simulink library "DRC_SimulinkLibrary"  (R2024a)
settings: Solver=VariableStepAuto  StartTime=0.0  StopTime=10.0  RelTol=1e-3
values from neighbouring files (symbols this model uses):
  T = 0.5*rho*A*R*V^2*Cp/TSR    [aerodynamictorque.m]
undefined symbols (not defined in the file or in its folder): DiscIntNeverNeededParam, freq, maxSatValue, OmegaVector, Ts, Wr0, WSE
libraries: $bdroot x16, spsEdgeDetectorLib x1
settings Model: Creator=Sebastiaan  LastModifiedBy=glazzerini
settings DebuggingCC: UnconnectedInputMsg=warning  UnconnectedOutputMsg=warning  UnconnectedLineMsg=warning
settings ModelReferenceCC: EnableRefExpFcnMdlSchedulingChecks=on
settings RTWCC: GPUComputeCapability=3.5  DLArmComputeVersion=19.05

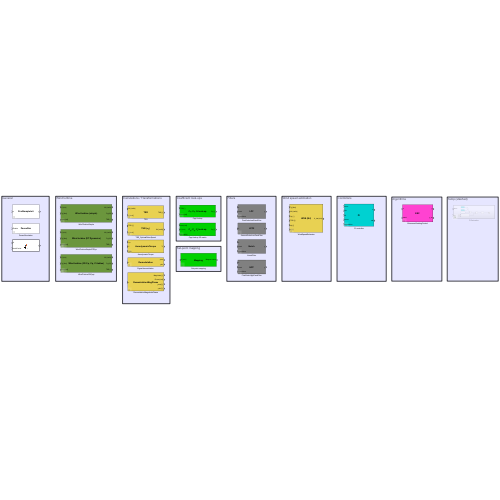
[thumbnail: Simulink's stored preview of the top-level diagram]
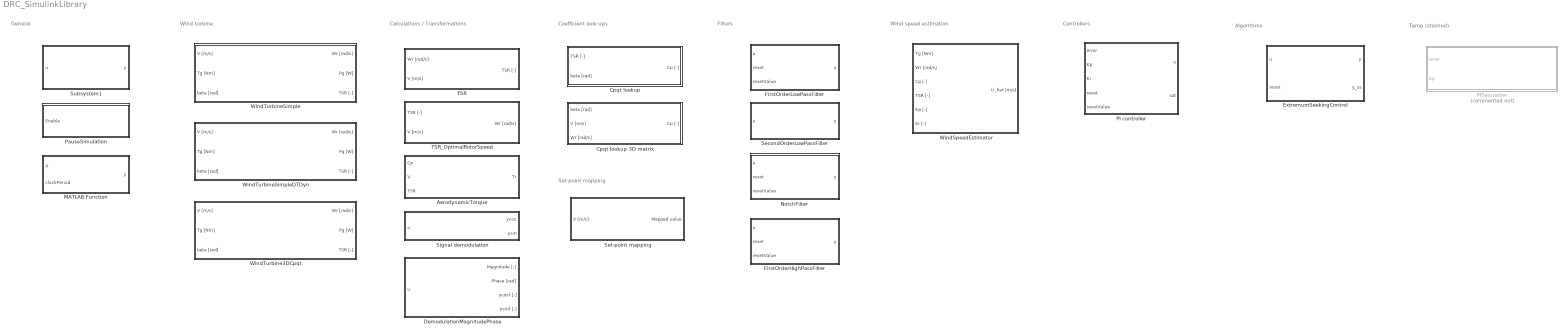
== system DRC_SimulinkLibrary ==
  note: Filters
  note: Coefficient look-ups
  note: General
  note: Algorithms
  note: Wind speed estimation
  note: Controllers
  note: Calculations / Transformations
  note: Temp (stashed)
  note: Wind turbine
  note: Set-point mapping
  AerodynamicTorque : Subsystem  mask(Aerodynamic rotor torque){R=10, rho=1.225, TrMax=inf}
      mask prompts: R "Rotor radius [m]"; rho "Air density [kg/m^3]"; TrMax "Maximum aerodynamic torque [Nm]"
      mask help: Calculates aerodynamic rotor torque based on the rotor radius, air density, power coefficient, wind speed and tip-speed ratio.
      mask Display: disp('{\bf\fontsize{12}AerodynamicTorque}', 'texmode', 'on');
  Cpqt lookup : Subsystem  mask(Coefficient look-up){CpqtGrid=[], TSRVector=[], PitchVector=[]}
      mask prompts: CpqtGrid "Cp/Cq/Ct grid [-]"; TSRVector "TSR vector [-]"; PitchVector "Pitch vector [rad]"
      mask help: Coefficient look-up table for power coefficient (Cp), torque coefficient (Cq), and thrust coefficient (Ct). The TSR and Pitch data should be a 1-dimensional vector of sizes p and q, respectively. The provided coefficient matrix should be of size p x q.
      mask Display: disp('{\bf\fontsize{12}C_p, C_q, C_t look-up}', 'texmode', 'on');
  Cpqt lookup 3D matrix : Subsystem  mask(Coefficient look-up){CpqtGrid=[], PitchVector=[], WindSpeedVector=[], OmegaVector=[]}
      mask prompts: CpqtGrid "Cp/Cq/Ct grid [-]"; PitchVector "Pitch vector [rad]"; WindSpeedVector "Wind Speed vector [m/s]"; OmegaVector "Omega vector [rad/s]"
      mask help: Coefficient look-up matrices for power coefficient (Cp), torque coefficient (Cq), and thrust coefficient (Ct). The Pitch, Wind-speed and Omega data should be 1-dimensional vectors of sizes p, q and r respectively. The provided coefficient matrix should be of size p x q x r.
      mask Display: disp('{\bf\fontsize{12}C_p, C_q, C_t look-up}', 'texmode', 'on');
  DemodulationMagnitudePhase : Subsystem  mask(Signal demodulation (mag/phase){freq=-1, phase_offset=0, Ts=-1, betaNum=0.1, betaDen=10}
      mask prompts: freq "Frequency [rad/s]"; phase_offset "Phase offset [rad]"; Ts "Sampling time [s]"; betaNum "Damping numerator"; betaDen "Damping denominator"
      mask help: This block demodulates a specific frequency in the input signal and returns its magnitude and phase. The input signal should have a zero-mean, which can for example be accomplished by high-pass or band-pass filtering.
      mask DialogControl Container3 Prompt: Notch parameters
      mask Display: disp('{\bf\fontsize{12}DemodulationMagPhase}', 'texmode', 'on');
  ExtremumSeekingControl : Subsystem  mask(Extremum Seeking Control (ESC)){D_A=3e5, D_w=0.09, M_phi=-30/180*pi, Ki=1000, LPF_wc=0.1, HPF_wc=0.02, Ts=Ts}
      mask prompts: D_A "Dither amplitude"; D_w "Dither frequency [rad/s]"; M_phi "Demodulation phase offset [rad]"; Ki "Integrator gain"; LPF_wc "LPF cut-off frequency [rad/s]"; HPF_wc "HPF cut-in frequency [rad/s]"; Ts "Sampling time [s]"
      mask help: Extremum Seeking Control (ESC) is a filter-based algorithm that excites a system with a periodic signal to attain a local maximum as a function of the input signal. By periodic excitation, demodulation and filtering actions the output gradient is retrieved, and subject to time integration until the steady-state signal that maximizes (or minimizes) the system output is attained.
      mask Display: disp('{\bf\fontsize{12}ESC}', 'texmode', 'on');
  FirstOrderHighPassFilter : Subsystem  mask(First order high-pass filter){wc=-1, Ts=-1}
      mask prompts: wc "Cut-off frequency [rad/s]"; Ts "Sampling time [s]"
      mask help:
      | Discrete time notch filter (IIR), given in continuous time by:
      | G =  s / (s + wc)
      | with wc the cut-off frequency, and s the Laplace operator.
      |
      | Discretized using the bilinear transform (Tustin's method). The sampling time should be explicitly specified.
      mask Display: disp('{\bf\fontsize{12}HPF}', 'texmode', 'on');
  FirstOrderLowPassFilter : Subsystem  mask(First order low-pass filter){wc=-1, Ts=-1}
      mask prompts: wc "Cut-in frequency [rad/s]"; Ts "Sampling time [s]"
      mask help:
      | Discrete time first order low-pass filter (IIR), given in continuous time by:
      | G = wc / ( s + wc)
      | with wc the cut-off frequency, and s the Laplace operator.
      |
      | Discretized using the bilinear transform (Tustin's method). The sampling time should be explicitly specified.
      mask Display: disp('{\bf\fontsize{12}LPF}', 'texmode', 'on');
  MATLAB Function : MATLAB Function  TreatAsAtomicUnit=on
  NotchFilter : Subsystem  mask{wn=-1, betaNum=-1, betaDen=-1, Ts=-1}
      mask prompts: wn "Target frequency [rad/s]"; betaNum "Beta numerator [-]"; betaDen "Beta denominator [-]"; Ts "Sampling time [s]"
      mask help:
      | Discrete time notch filter (IIR), given in continuous time by:
      | G =  ( s^2 + 2*wc*betaNum*s + wc^2 ) / ( s^2 + 2*wc*betaDen*s + wc^2 )
      | with wc the cut-off frequency, betaNum and betaDen being the damping coefficients, and s the Laplace operator. The ratio and magnitude of the ratio determines the width and depth of the notch.
      |
      | Discretized using the bilinear transform (Tustin's method). The sampling time should be explicitly specified.
      mask Display: disp('{\bf\fontsize{12}Notch}', 'texmode', 'on');
  PI controller : Subsystem  mask(PI controller){minSatValue=0, maxSatValue=inf, Ts=Ts}
      mask prompts: minSatValue "Minimum saturation"; maxSatValue "Maximum saturation"; Ts "Sampling time [s]"
      mask help:
      | Proportional-Integral (PI) controller with saturation limits. The error port is the input to the controller, Kp and Ki are the proportional and integral gains amplifying the error signal. When reset is true, the integral state is reset to resetValue.
      |
      | The sat output port indicates whether the controller is saturated or if the reset port is true.
      mask Display: disp('{\bf\fontsize{12}PI}', 'texmode', 'on');
  PISaturation : Subsystem  Commented=on
  PauseSimulation : Subsystem  mask(Pause simulation){PauseEach=0.5, Ts=Ts}
      mask prompts: PauseEach "Pause each [s]"; Ts "Sampling time [s]"
      mask help: Pause simulation after integer multiples of the specified value.
      mask Display: disp('{\bf\fontsize{12}PauseSim}', 'texmode', 'on');
  SecondOrderLowPassFilter : Subsystem  mask(Second order low-pass filter){wn=-1, damp=-1, Ts=-1}
      mask prompts: wn "Cut-off frequency [rad/s]"; damp "Damping coefficient [-]"; Ts "Sampling time [s]"
      mask help:
      | Discrete time second order low-pass filter (IIR), given in continuous time by:
      | G = wc^2 / ( s^2 + 2*wc*zeta*s + wc^2)
      | with wc the cut-off frequency, zeta the damping coefficient, and s the Laplace operator.
      |
      | Discretized using the bilinear transform (Tustin's method). The sampling time should be explicitly specified.
      mask Display: disp('{\bf\fontsize{12}LPF2}', 'texmode', 'on');
  Set-point mapping : Subsystem  mask(Mapping look-up){MappingVector=[], WindSpeedVector=[]}
      mask help: Mapping look-up for rotational speed or collective pitch angle vs windspeed. The input data should be a 1-dimensional value. The provided value will represent the mapping.
      mask Display: disp('{\bf\fontsize{12}Mapping}', 'texmode', 'on');
  "Signal demodulation " : Subsystem  mask(Signal demodulation){freq=freq, phase_offset=0, Ts=Ts}
      mask prompts: freq "Frequency [rad/s]"; phase_offset "Phase offset [rad]"; Ts "Sampling time [s]"
      mask help: This block demodulates a specific frequency in the input signal and returns the sine and cosine projections as output. The input signal should have a zero-mean, which can for example be accomplished by high-pass or band-pass filtering.
      mask Display: disp('{\bf\fontsize{12}Demodulation}', 'texmode', 'on');
  Subsystem1 : Subsystem  mask(First sample initialization){u_init=0}
      mask prompts: u_init "First sample"
      mask help: Returns the value specified by First sample in the very first time step. In subsequent time steps: y=u.
      mask Display: disp('{\bf\fontsize{12}FirstSampleInit}', 'texmode', 'on');
  TSR : Subsystem  mask(Tip-speed ratio){RotorRadius=10}
      mask prompts: RotorRadius "Rotor radius [m]"
      mask help: Calculates the tip-speed ratio based on rotor speed [rad/s] and wind speed [m/s] signals.
      mask Display: disp('{\bf\fontsize{12}TSR}', 'texmode', 'on');
  TSR_OptimalRotorSpeed : Subsystem  mask(Tip-speed ratio (rotor speed)){RotorRadius=10}
      mask prompts: RotorRadius "Rotor radius [m]"
      mask help: Calculates the corresponding rotor speed [rad/s] based on tip-speed ratio [-] and wind speed [m/s] signals.
      mask Display: disp('{\bf\fontsize{12}TSR (\omega_r)}', 'texmode', 'on');
  WindSpeedEstimator : Subsystem  mask(Wind speed estimator (I&I)){R=T.R, TrMax=T.Tgen_max*T.G, G=T.G, JLss=T.Jlss, rho=T.rho, omega_r_0=WSE.omega_r_0, V0=0, Ts=Ts}
      mask prompts: R "Rotor radius [m]"; TrMax "Max. exp. rotor torque [Nm]"; G "Gearbox ratio"; JLss "Drivetrain inertia (LSS)"; rho "Air density [kg/m^3]"; omega_r_0 "Rotor speed initial condition"; V0 "Wind speed initial condition"; Ts "Sampling time [s]"
      mask help: Immersion and Invariance (I&I) wind speed estimator. Uses prior power coefficient information of the turbine to obtain an estimate of the aerodynamic rotor torque. Together with the measured generator torque and rotor speed, an estimate of the wind speed is computed.
      mask Display: disp('{\bf\fontsize{12}WSE (I&I)}', 'texmode', 'on');
  WindTurbine3DCpqt : Subsystem  AncestorBlock=DRC_SimulinkLibrary/WindTurbineSimple  mask{R=T.R, rho=T.rho, TMax=inf, JWr=T.Jlss, G=T.G, Wr0=Wr0, CpArray=T.Cp, betaVec=T.CPitch, wsVec=T.CWindSpeed, omegaVec=T.COmega}
      mask prompts: R "Rotor radius [m]"; rho "Air density [kg/m^3]"; TMax "Maximum aerodynamic torque [Nm]"; JWr "Inertia low-speed shaft [kg m^2]"; G "Gearbox ratio [-]"; Wr0 "Rotor speed initial condition [rad/s]"; CpArray "Cp matrix"; betaVec "Pitch vector [rad]"; wsVec "Wind speed vector [m/s]"; omegaVec "Omega vector [rad/s]"
      mask DialogControl CpGroupVar Prompt: Power coefficient (Cp)
      mask Display: disp('{\bf\fontsize{12}Wind turbine (3D Cp, Cq, Ct tables)}', 'texmode', 'on');
  WindTurbineSimple : Subsystem  mask{R=T.R, rho=T.rho, TMax=inf, JWr=T.Jlss, G=T.G, Wr0=Wr0, CpArray=T.Cp, TSRVec=T.CTSR, betaVec=T.CPitch}
      mask prompts: R "Rotor radius [m]"; rho "Air density [kg/m^3]"; TMax "Maximum aerodynamic torque [Nm]"; JWr "Inertia low-speed shaft [kg m^2]"; G "Gearbox ratio [-]"; Wr0 "Rotor speed initial condition [rad/s]"; CpArray "Cp matrix"; TSRVec "Tip-speed ratio vector"; betaVec "Pitch vector [rad]"
      mask DialogControl CpGroupVar Prompt: Power coefficient (Cp)
      mask Display: disp('{\bf\fontsize{12}Wind turbine (simple)}', 'texmode', 'on');
  WindTurbineSimpleDTDyn : Subsystem  AncestorBlock=DRC_SimulinkLibrary/WindTurbineSimple  mask{R=T.R, rho=T.rho, TMax=inf, JWr=3*T.Jb + T.Jh, JWg=T.Jg, G=T.G, Wr0=Wr0, ks=T.k_dt, bs=T.c_dt, CpArray=T.Cp, TSRVec=T.CTSR, betaVec=T.CPitch}
      mask prompts: R "Rotor radius [m]"; rho "Air density [kg/m^3]"; TMax "Maximum aerodynamic torque [Nm]"; JWr "Inertia rotor [kg m^2]"; JWg "Inertia generator [kg m^2]"; G "Gearbox ratio [-] UNUSED!!"; Wr0 "Rotor speed initial condition [rad/s]"; ks "Spring constant [Nm/rad]"; bs "Damping coefficient [N-m/(rad/s)]"; CpArray "Cp matrix"; TSRVec "Tip-speed ratio vector"; betaVec "Pitch vector [rad]"
      mask help: NOTE: Be sure to sample with a low sampling time to avoid numerical instabilities (order 1e-3)
      mask DialogControl Container4 Prompt: Drivetrain
      mask DialogControl CpGroupVar Prompt: Power coefficient (Cp)
      mask Display: disp('{\bf\fontsize{12}Wind turbine (DT Dynamics)}', 'texmode', 'on');

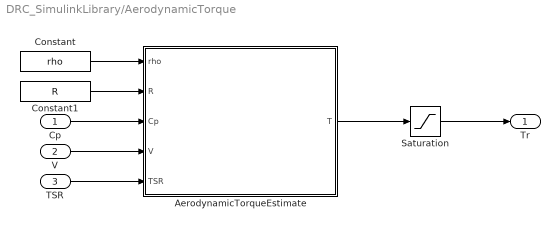
== system DRC_SimulinkLibrary/AerodynamicTorque ==
  Cp : Inport
  V : Inport  Port=2
  TSR : Inport  Port=3
  AerodynamicTorqueEstimate : MATLAB Function  TreatAsAtomicUnit=on
  Constant : Constant  Value=rho
  Constant1 : Constant  Value=R
  Saturation : Saturate  UpperLimit=TrMax  LowerLimit=0
  Tr : Outport
  wires:
  Constant/1 -> AerodynamicTorqueEstimate/1(rho)
  V/1 -> AerodynamicTorqueEstimate/4(V)
  AerodynamicTorqueEstimate/1(T) -> Saturation/1
  Cp/1 -> AerodynamicTorqueEstimate/3(Cp)
  TSR/1 -> AerodynamicTorqueEstimate/5(TSR)
  Constant1/1 -> AerodynamicTorqueEstimate/2(R)
  Saturation/1 -> Tr/1

== system DRC_SimulinkLibrary/Cpqt lookup ==
  TSR [-] : Inport
  beta [rad] : Inport  Port=2
  CP lookup : Lookup_n-D  BreakpointsForDimension1=TSRVector  BreakpointsForDimension2=PitchVector  Table=CpqtGrid  InternalRulePriority=Speed  RndMeth=Simplest
      settings: InputPortMap=u0,u1
  Saturation : Saturate  UpperLimit=1.0  LowerLimit=eps
  Cp [-] : Outport
  wires:
  beta [rad]/1 -> CP lookup/2
  TSR [-]/1 -> CP lookup/1
  CP lookup/1 -> Saturation/1
  Saturation/1 -> Cp [-]/1

== system DRC_SimulinkLibrary/Cpqt lookup 3D matrix ==
  beta [rad] : Inport
  V [m/s] : Inport  Port=2
  Wr [rad/s] : Inport  Port=3
  CP lookup : Lookup_n-D  NumberOfTableDimensions=3  BreakpointsForDimension1=PitchVector  BreakpointsForDimension2=WindSpeedVector  BreakpointsForDimension3=OmegaVector  Table=CpqtGrid  InternalRulePriority=Speed  RndMeth=Simplest
      settings: InputPortMap=u0,u1,u2
  Saturation : Saturate  UpperLimit=1.0  LowerLimit=eps
  Cp [-] : Outport
  wires:
  Saturation/1 -> Cp [-]/1
  CP lookup/1 -> Saturation/1
  V [m/s]/1 -> CP lookup/2
  Wr [rad/s]/1 -> CP lookup/3
  beta [rad]/1 -> CP lookup/1

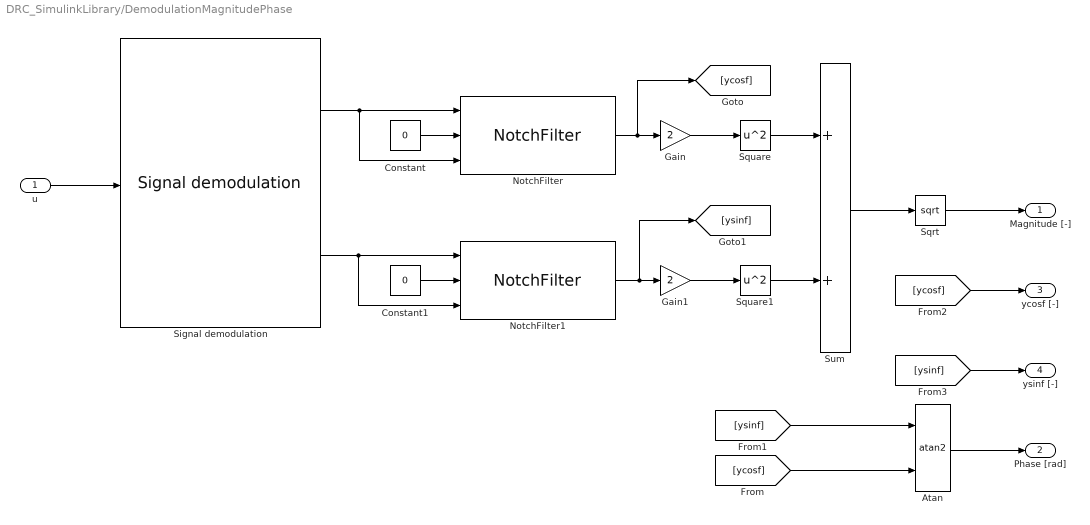
== system DRC_SimulinkLibrary/DemodulationMagnitudePhase ==
  u : Inport
  Atan : Trigonometry  Operator=atan2
  Constant : Constant  Value=0
  Constant1 : Constant  Value=0
  Gain : Gain  Gain=2
  Gain1 : Gain  Gain=2
  NotchFilter : $bdroot/NotchFilter  wn=2*freq  betaNum=betaNum  betaDen=betaDen  Ts=Ts
  NotchFilter1 : $bdroot/NotchFilter  wn=2*freq  betaNum=betaNum  betaDen=betaDen  Ts=Ts
  "Signal demodulation " : $bdroot/Signal demodulation   freq=freq  phase_offset=phase_offset  Ts=Ts
  Sqrt : Sqrt
  Square : Math  Operator=square
  Square1 : Math  Operator=square
  Sum : Sum
  Magnitude [-] : Outport
  Phase [rad] : Outport  Port=2
  ycosf [-] : Outport  Port=3
  ysinf [-] : Outport  Port=4
  wires:
  "Signal demodulation "/1 -> NotchFilter/3, NotchFilter/1
  "Signal demodulation "/2 -> NotchFilter1/3, NotchFilter1/1
  NotchFilter/1 -> [ycosf], Gain/1
  Constant/1 -> NotchFilter/2
  u/1 -> "Signal demodulation "/1
  Atan/1 -> Phase [rad]/1
  Constant1/1 -> NotchFilter1/2
  Sqrt/1 -> Magnitude [-]/1
  Square1/1 -> Sum/2
  NotchFilter1/1 -> [ysinf], Gain1/1
  Square/1 -> Sum/1
  Gain/1 -> Square/1
  Sum/1 -> Sqrt/1
  Gain1/1 -> Square1/1
  [ysinf] -> Atan/1
  [ycosf] -> Atan/2
  [ycosf] -> ycosf [-]/1
  [ysinf] -> ysinf [-]/1

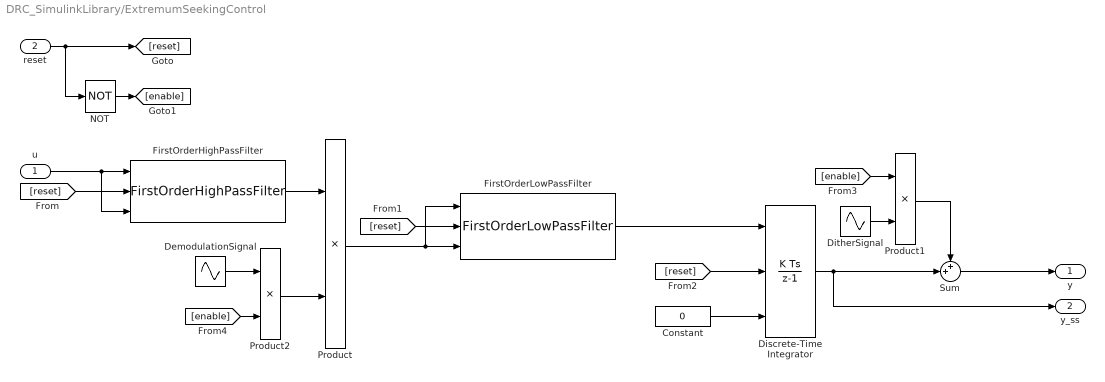
== system DRC_SimulinkLibrary/ExtremumSeekingControl ==
  u : Inport
  reset : Inport  Port=2
  Constant : Constant  Value=0
  DemodulationSignal : Sin  Amplitude=2/D_A  Frequency=D_w  Phase=M_phi  SampleTime=Ts
  Discrete-Time Integrator : DiscreteIntegrator  gainval=Ki  ExternalReset=level  InitialConditionSource=external  SampleTime=Ts  ICPrevOutput=DiscIntNeverNeededParam  ICPrevScaledInput=DiscIntNeverNeededParam
  DitherSignal : Sin  Amplitude=D_A  Frequency=D_w  SampleTime=Ts
  FirstOrderHighPassFilter : $bdroot/FirstOrderHighPassFilter  wc=HPF_wc  Ts=Ts
  FirstOrderLowPassFilter : $bdroot/FirstOrderLowPassFilter  wc=LPF_wc  Ts=Ts
  NOT : Logic  Operator=NOT  IconShape=distinctive  AllPortsSameDT=off  OutDataTypeStr=boolean
  Product : Product
  Product1 : Product
  Product2 : Product
  Sum : Sum  Inputs=++|
  y : Outport
  y_ss : Outport  Port=2
  wires:
  [enable] -> Product2/2
  Product2/1 -> Product/2
  [enable] -> Product1/1
  NOT/1 -> [enable]
  Product1/1 -> Sum/1
  DitherSignal/1 -> Product1/2
  Constant/1 -> Discrete-Time Integrator/3
  [reset] -> Discrete-Time Integrator/2
  reset/1 -> [reset], NOT/1
  u/1 -> FirstOrderHighPassFilter/3, FirstOrderHighPassFilter/1
  FirstOrderLowPassFilter/1 -> Discrete-Time Integrator/1
  DemodulationSignal/1 -> Product2/1
  [reset] -> FirstOrderLowPassFilter/2
  Discrete-Time Integrator/1 -> Sum/2, y_ss/1
  Product/1 -> FirstOrderLowPassFilter/3, FirstOrderLowPassFilter/1
  FirstOrderHighPassFilter/1 -> Product/1
  [reset] -> FirstOrderHighPassFilter/2
  Sum/1 -> y/1

== system DRC_SimulinkLibrary/FirstOrderHighPassFilter ==
  u : Inport
  reset : Inport  Port=2
  resetValue : Inport  Port=3
  Constant : Constant  Value=wc
  Constant1 : Constant  Value=Ts
  HighPassFilter : MATLAB Function  TreatAsAtomicUnit=on
  y : Outport
  wires:
  HighPassFilter/1(y) -> y/1
  reset/1 -> HighPassFilter/3(reset)
  Constant/1 -> HighPassFilter/2(wc)
  Constant1/1 -> HighPassFilter/5(Ts)
  u/1 -> HighPassFilter/1(u)
  resetValue/1 -> HighPassFilter/4(resetValue)

== system DRC_SimulinkLibrary/FirstOrderLowPassFilter ==
  u : Inport
  reset : Inport  Port=2
  resetValue : Inport  Port=3
  Constant : Constant  Value=wc
  Constant1 : Constant  Value=Ts
  First-order low-pass filter : MATLAB Function  TreatAsAtomicUnit=on
  y : Outport
  wires:
  resetValue/1 -> First-order low-pass filter/4(resetValue)
  First-order low-pass filter/1(y) -> y/1
  reset/1 -> First-order low-pass filter/3(reset)
  Constant/1 -> First-order low-pass filter/2(wc)
  Constant1/1 -> First-order low-pass filter/5(Ts)
  u/1 -> First-order low-pass filter/1(u)

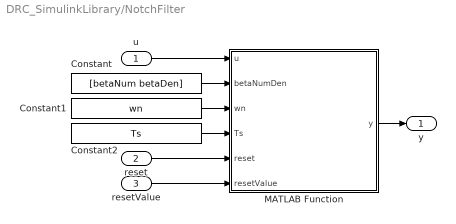
== system DRC_SimulinkLibrary/NotchFilter ==
  u : Inport
  reset : Inport  Port=2
  resetValue : Inport  Port=3
  Constant : Constant  Value=[betaNum betaDen]
  Constant1 : Constant  Value=wn
  Constant2 : Constant  Value=Ts
  MATLAB Function : MATLAB Function  TreatAsAtomicUnit=on
  y : Outport
  wires:
  Constant1/1 -> MATLAB Function/3(wn)
  MATLAB Function/1(y) -> y/1
  Constant2/1 -> MATLAB Function/4(Ts)
  Constant/1 -> MATLAB Function/2(betaNumDen)
  u/1 -> MATLAB Function/1(u)
  reset/1 -> MATLAB Function/5(reset)
  resetValue/1 -> MATLAB Function/6(resetValue)

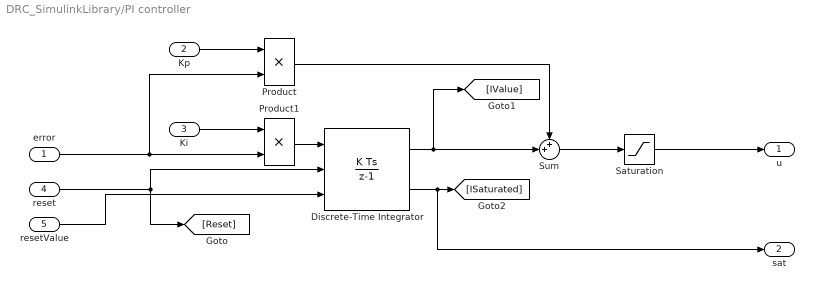
== system DRC_SimulinkLibrary/PI controller ==
  error : Inport
  Kp : Inport  Port=2
  Ki : Inport  Port=3
  reset : Inport  Port=4
  resetValue : Inport  Port=5
  Discrete-Time Integrator : DiscreteIntegrator  ExternalReset=level  InitialConditionSource=external  SampleTime=Ts  LimitOutput=on  UpperSaturationLimit=maxSatValue  LowerSaturationLimit=minSatValue  ShowSaturationPort=on  ICPrevOutput=DiscIntNeverNeededParam  ICPrevScaledInput=DiscIntNeverNeededParam
  Product : Product
  Product1 : Product
  Saturation : Saturate  UpperLimit=maxSatValue  LowerLimit=minSatValue
  Sum : Sum  Inputs=++|
  u : Outport
  sat : Outport  Port=2
  wires:
  Product/1 -> Sum/1
  resetValue/1 -> Discrete-Time Integrator/3
  reset/1 -> Discrete-Time Integrator/2, [Reset]
  Kp/1 -> Product/1
  Saturation/1 -> u/1
  Discrete-Time Integrator/1 -> [IValue], Sum/2
  error/1 -> Product1/2, Product/2
  Product1/1 -> Discrete-Time Integrator/1
  Ki/1 -> Product1/1
  Sum/1 -> Saturation/1
  Discrete-Time Integrator/2 -> [ISaturated], sat/1

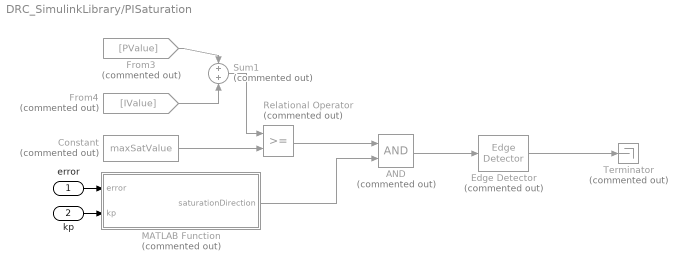
== system DRC_SimulinkLibrary/PISaturation ==
  error : Inport
  kp : Inport  Port=2
  AND : Logic  Commented=on  AllPortsSameDT=off  OutDataTypeStr=boolean
  Constant : Constant  Commented=on  Value=maxSatValue
  Edge Detector : spsEdgeDetectorLib/Edge Detector  Commented=on  model=Rising  ic=0  Ts=0
  From3 : From  Commented=on  GotoTag=PValue
  From4 : From  Commented=on  GotoTag=IValue
  MATLAB Function : MATLAB Function  Commented=on  TreatAsAtomicUnit=on
  Relational Operator : RelationalOperator  Commented=on  OutDataTypeStr=boolean  RndMeth=Simplest  InputSameDT=off
  Sum1 : Sum  Commented=on
  Terminator : Terminator  Commented=on
  wires:
  Relational Operator/1 -> AND/1
  Sum1/1 -> Relational Operator/1
  Constant/1 -> Relational Operator/2
  Edge Detector/1 -> Terminator/1
  From4/1 -> Sum1/2
  AND/1 -> Edge Detector/1
  From3/1 -> Sum1/1
  MATLAB Function/1(saturationDirection) -> AND/2
  error/1 -> MATLAB Function/1(error)
  kp/1 -> MATLAB Function/2(kp)

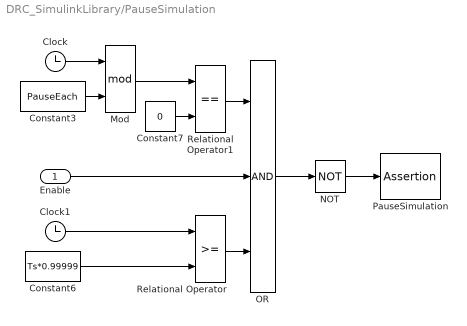
== system DRC_SimulinkLibrary/PauseSimulation ==
  Enable : Inport
  Clock : Clock
  Clock1 : Clock
  Constant3 : Constant  Value=PauseEach
  Constant6 : Constant  Value=Ts*0.99999
  Constant7 : Constant  Value=0
  Mod : Math  Operator=mod  SignedPower=on
  NOT : Logic  Operator=NOT  IconShape=distinctive  AllPortsSameDT=off  OutDataTypeStr=boolean
  OR : Logic  Inputs=3  AllPortsSameDT=off  OutDataTypeStr=boolean
  PauseSimulation : Assertion  AssertionFailFcn=set_param(bdroot,'SimulationCommand','pause')  StopWhenAssertionFail=off
  Relational Operator : RelationalOperator  OutDataTypeStr=boolean  RndMeth=Simplest  InputSameDT=off
  Relational Operator1 : RelationalOperator  Operator===  OutDataTypeStr=boolean  ZeroCross=off  RndMeth=Simplest  InputSameDT=off
  wires:
  Relational Operator/1 -> OR/3
  Constant6/1 -> Relational Operator/2
  Clock1/1 -> Relational Operator/1
  NOT/1 -> PauseSimulation/1
  Mod/1 -> Relational Operator1/1
  Clock/1 -> Mod/1
  Constant3/1 -> Mod/2
  Relational Operator1/1 -> OR/1
  OR/1 -> NOT/1
  Constant7/1 -> Relational Operator1/2
  Enable/1 -> OR/2

== system DRC_SimulinkLibrary/SecondOrderLowPassFilter ==
  u : Inport
  Constant : Constant  Value=Ts
  Constant1 : Constant  Value=damp
  Constant2 : Constant  Value=wn
  Second-order low-pass filter : MATLAB Function  TreatAsAtomicUnit=on
  y : Outport
  wires:
  u/1 -> Second-order low-pass filter/1(u)
  Constant2/1 -> Second-order low-pass filter/2(wn)
  Second-order low-pass filter/1(y) -> y/1
  Constant1/1 -> Second-order low-pass filter/3(Damp)
  Constant/1 -> Second-order low-pass filter/4(Ts)

== system DRC_SimulinkLibrary/Set-point mapping ==
  V [m/s] : Inport
  Saturation : Saturate  UpperLimit=1.0  LowerLimit=eps
  f(V) : Lookup_n-D  NumberOfTableDimensions=1  BreakpointsForDimension1=WindSpeedVector  BreakpointsForDimension2=WindSpeedVector  BreakpointsForDimension3=OmegaVector  Table=MappingVector  InternalRulePriority=Speed  RndMeth=Simplest
  Mapped value : Outport
  wires:
  Saturation/1 -> Mapped value/1
  f(V)/1 -> Saturation/1
  V [m/s]/1 -> f(V)/1

== system DRC_SimulinkLibrary/Signal demodulation  ==
  u : Inport
  Cos : Sin  Frequency=freq  Phase=pi/2+phase_offset  SampleTime=Ts
  Product1 : Product  RndMeth=Zero
  Product4 : Product  RndMeth=Zero
  Sin : Sin  Frequency=freq  Phase=phase_offset  SampleTime=Ts
  ycos : Outport  VectorParamsAs1DForOutWhenUnconnected=off
  ysin : Outport  Port=2  VectorParamsAs1DForOutWhenUnconnected=off
  wires:
  Product4/1 -> ysin/1
  Product1/1 -> ycos/1
  u/1 -> Product4/1, Product1/1
  Sin/1 -> Product4/2
  Cos/1 -> Product1/2

== system DRC_SimulinkLibrary/Subsystem1 ==
  u : Inport
  Constant : Constant  Value=u_init
  MATLAB Function : MATLAB Function  TreatAsAtomicUnit=on
  y : Outport
  wires:
  MATLAB Function/1(y) -> y/1
  Constant/1 -> MATLAB Function/2(u_init)
  u/1 -> MATLAB Function/1(u)

== system DRC_SimulinkLibrary/TSR ==
  Wr [rad/s] : Inport
  V [m/s] : Inport  Port=2
  Constant : Constant  Value=RotorRadius
  Mux : Mux  Inputs=3
  TSR : MATLAB Function  TreatAsAtomicUnit=on
  TSR [-] : Outport
  wires:
  Constant/1 -> Mux/3
  Mux/1 -> TSR/1(u)
  V [m/s]/1 -> Mux/2
  Wr [rad/s]/1 -> Mux/1
  TSR/1(tsr_out) -> TSR [-]/1

== system DRC_SimulinkLibrary/TSR_OptimalRotorSpeed ==
  TSR [-] : Inport
  V [m/s] : Inport  Port=2
  Constant : Constant  Value=RotorRadius
  Mux : Mux  Inputs=3
  Optimal rotor speed : MATLAB Function  TreatAsAtomicUnit=on
  Wr [rad/s] : Outport
  wires:
  Optimal rotor speed/1(Wr_opt) -> Wr [rad/s]/1
  V [m/s]/1 -> Mux/2
  Mux/1 -> Optimal rotor speed/1(u)
  Constant/1 -> Mux/3
  TSR [-]/1 -> Mux/1

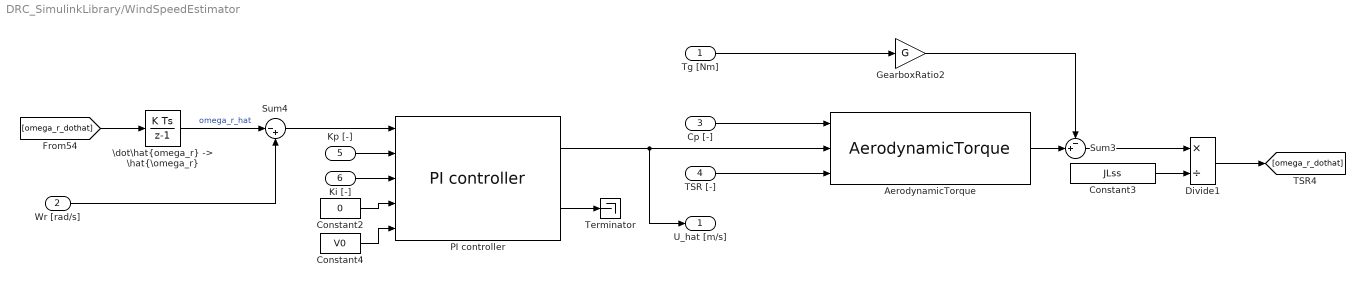
== system DRC_SimulinkLibrary/WindSpeedEstimator ==
  Tg [Nm] : Inport
  Wr [rad/s] : Inport  Port=2
  Cp [-] : Inport  Port=3
  TSR [-] : Inport  Port=4
  Kp [-] : Inport  Port=5
  Ki [-] : Inport  Port=6
  AerodynamicTorque : $bdroot/AerodynamicTorque  R=R  rho=rho  TrMax=TrMax
  Constant2 : Constant  Value=0
  Constant3 : Constant  Value=JLss
  Constant4 : Constant  Value=V0
  Divide1 : Product  Inputs=*/
  GearboxRatio2 : Gain  Gain=G
  PI controller : $bdroot/PI controller  minSatValue=0  maxSatValue=inf  Ts=Ts
  Sum3 : Sum  Inputs=-+|
  Sum4 : Sum  Inputs=|-+
  Terminator : Terminator
  "\\dot\\hat{omega_r} -> \\hat{\\omega_r}" : DiscreteIntegrator  InitialCondition=omega_r_0  SampleTime=Ts  ICPrevOutput=DiscIntNeverNeededParam  ICPrevScaledInput=DiscIntNeverNeededParam
  U_hat [m/s] : Outport
  wires:
  PI controller/1 -> U_hat [m/s]/1, AerodynamicTorque/2
  Divide1/1 -> [omega_r_dothat]
  AerodynamicTorque/1 -> Sum3/2
  "\\dot\\hat{omega_r} -> \\hat{\\omega_r}"/1 -> Sum4/1  "omega_r_hat"
  GearboxRatio2/1 -> Sum3/1
  Constant3/1 -> Divide1/2
  Sum3/1 -> Divide1/1
  [omega_r_dothat] -> "\\dot\\hat{omega_r} -> \\hat{\\omega_r}"/1
  Tg [Nm]/1 -> GearboxRatio2/1
  Wr [rad/s]/1 -> Sum4/2
  Cp [-]/1 -> AerodynamicTorque/1
  TSR [-]/1 -> AerodynamicTorque/3
  Sum4/1 -> PI controller/1
  Kp [-]/1 -> PI controller/2
  Ki [-]/1 -> PI controller/3
  Constant2/1 -> PI controller/4
  Constant4/1 -> PI controller/5
  PI controller/2 -> Terminator/1

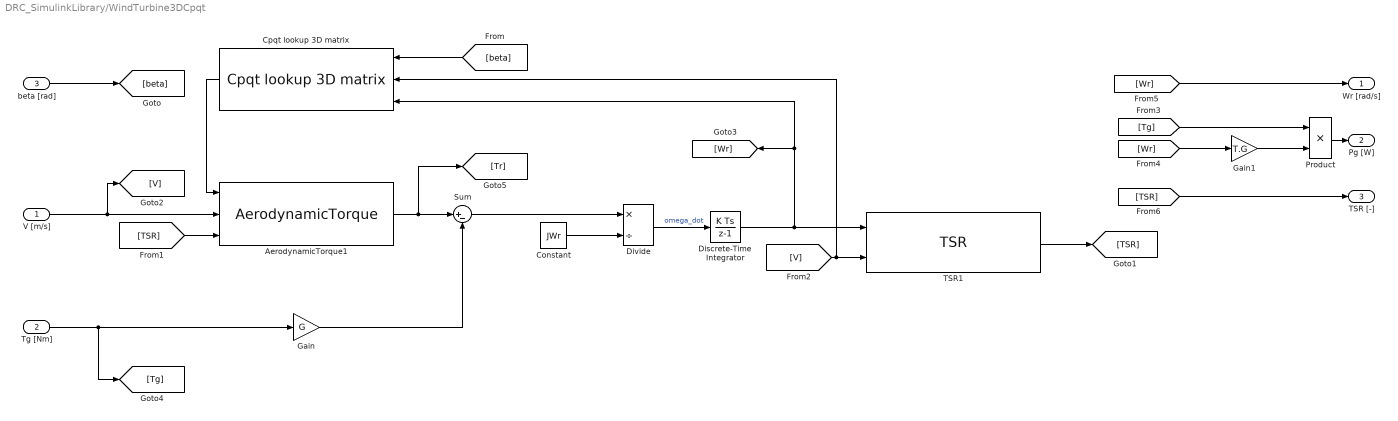
== system DRC_SimulinkLibrary/WindTurbine3DCpqt ==
  V [m/s] : Inport
  Tg [Nm] : Inport  Port=2
  beta [rad] : Inport  Port=3
  AerodynamicTorque1 : $bdroot/AerodynamicTorque  R=R  rho=rho  TrMax=TMax
  Constant : Constant  Value=JWr
  Cpqt lookup 3D matrix : $bdroot/Cpqt lookup 3D matrix  CpqtGrid=CpArray  PitchVector=betaVec  WindSpeedVector=wsVec  OmegaVector=omegaVec
  Discrete-Time Integrator : DiscreteIntegrator  InitialCondition=Wr0  SampleTime=-1  ICPrevOutput=DiscIntNeverNeededParam  ICPrevScaledInput=DiscIntNeverNeededParam
  Divide : Product  Inputs=*/
  Gain : Gain  Gain=G
  Gain1 : Gain  Gain=T.G
  Product : Product
  Sum : Sum  Inputs=|+-
  TSR1 : $bdroot/TSR  RotorRadius=R
  Wr [rad/s] : Outport
  Pg [W] : Outport  Port=2
  TSR [-] : Outport  Port=3
  wires:
  [TSR] -> AerodynamicTorque1/3
  Gain/1 -> Sum/2
  Tg [Nm]/1 -> Gain/1, [Tg]
  beta [rad]/1 -> [beta]
  Constant/1 -> Divide/2
  V [m/s]/1 -> [V], AerodynamicTorque1/2
  [beta] -> Cpqt lookup 3D matrix/1
  Divide/1 -> Discrete-Time Integrator/1  "omega_dot"
  Discrete-Time Integrator/1 -> Cpqt lookup 3D matrix/3, [Wr], TSR1/1
  AerodynamicTorque1/1 -> [Tr], Sum/1
  Sum/1 -> Divide/1
  TSR1/1 -> [TSR]
  [V] -> Cpqt lookup 3D matrix/2, TSR1/2
  Gain1/1 -> Product/2
  Product/1 -> Pg [W]/1
  [Wr] -> Gain1/1
  [Tg] -> Product/1
  [Wr] -> Wr [rad/s]/1
  [TSR] -> TSR [-]/1
  Cpqt lookup 3D matrix/1 -> AerodynamicTorque1/1

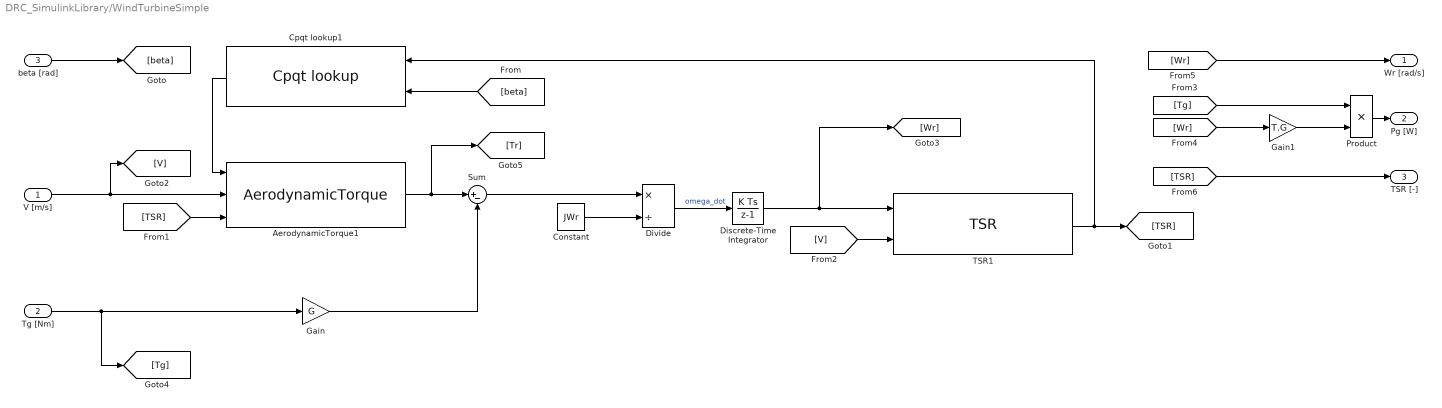
== system DRC_SimulinkLibrary/WindTurbineSimple ==
  V [m/s] : Inport
  Tg [Nm] : Inport  Port=2
  beta [rad] : Inport  Port=3
  AerodynamicTorque1 : $bdroot/AerodynamicTorque  R=R  rho=rho  TrMax=TMax
  Constant : Constant  Value=JWr
  Cpqt lookup1 : $bdroot/Cpqt lookup  CpqtGrid=CpArray  TSRVector=TSRVec  PitchVector=betaVec
  Discrete-Time Integrator : DiscreteIntegrator  InitialCondition=Wr0  SampleTime=-1  ICPrevOutput=DiscIntNeverNeededParam  ICPrevScaledInput=DiscIntNeverNeededParam
  Divide : Product  Inputs=*/
  Gain : Gain  Gain=G
  Gain1 : Gain  Gain=T.G
  Product : Product
  Sum : Sum  Inputs=|+-
  TSR1 : $bdroot/TSR  RotorRadius=R
  Wr [rad/s] : Outport
  Pg [W] : Outport  Port=2
  TSR [-] : Outport  Port=3
  wires:
  [TSR] -> AerodynamicTorque1/3
  Gain/1 -> Sum/2
  Tg [Nm]/1 -> Gain/1, [Tg]
  beta [rad]/1 -> [beta]
  Constant/1 -> Divide/2
  V [m/s]/1 -> [V], AerodynamicTorque1/2
  [beta] -> Cpqt lookup1/2
  Cpqt lookup1/1 -> AerodynamicTorque1/1
  Divide/1 -> Discrete-Time Integrator/1  "omega_dot"
  Discrete-Time Integrator/1 -> [Wr], TSR1/1
  AerodynamicTorque1/1 -> [Tr], Sum/1
  Sum/1 -> Divide/1
  TSR1/1 -> Cpqt lookup1/1, [TSR]
  [V] -> TSR1/2
  Gain1/1 -> Product/2
  Product/1 -> Pg [W]/1
  [Wr] -> Gain1/1
  [Tg] -> Product/1
  [Wr] -> Wr [rad/s]/1
  [TSR] -> TSR [-]/1

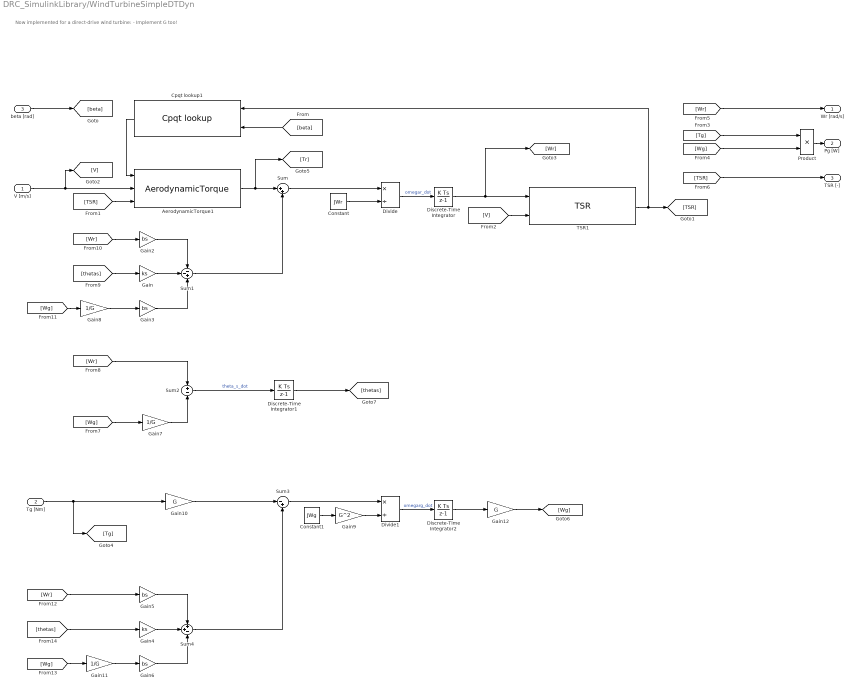
== system DRC_SimulinkLibrary/WindTurbineSimpleDTDyn ==
  note: Now implemented for a direct-drive wind turbine:
      | - Implement G too!
  V [m/s] : Inport
  Tg [Nm] : Inport  Port=2
  beta [rad] : Inport  Port=3
  AerodynamicTorque1 : $bdroot/AerodynamicTorque  R=R  rho=rho  TrMax=TMax
  Constant : Constant  Value=JWr
  Constant1 : Constant  Value=JWg
  Cpqt lookup1 : $bdroot/Cpqt lookup  CpqtGrid=CpArray  TSRVector=TSRVec  PitchVector=betaVec
  Discrete-Time Integrator : DiscreteIntegrator  InitialCondition=Wr0  SampleTime=-1  ICPrevOutput=DiscIntNeverNeededParam  ICPrevScaledInput=DiscIntNeverNeededParam
  Discrete-Time Integrator1 : DiscreteIntegrator  SampleTime=-1  ICPrevOutput=DiscIntNeverNeededParam  ICPrevScaledInput=DiscIntNeverNeededParam
  Discrete-Time Integrator2 : DiscreteIntegrator  InitialCondition=Wr0  SampleTime=-1  ICPrevOutput=DiscIntNeverNeededParam  ICPrevScaledInput=DiscIntNeverNeededParam
  Divide : Product  Inputs=*/
  Divide1 : Product  Inputs=*/
  Gain : Gain  Gain=ks
  Gain10 : Gain  Gain=G
  Gain11 : Gain  Gain=1/G
  Gain12 : Gain  Gain=G
  Gain{2..3,5..6} (4 alike) : Gain  Gain=bs
  Gain4 : Gain  Gain=ks
  Gain7 : Gain  Gain=1/G
  Gain8 : Gain  Gain=1/G
  Gain9 : Gain  Gain=G^2
  Product : Product
  Sum : Sum  Inputs=|++
  Sum1 : Sum  Inputs=--+
  Sum2 : Sum  Inputs=+-
  Sum3 : Sum  Inputs=|-+
  Sum4 : Sum  Inputs=++-
  TSR1 : $bdroot/TSR  RotorRadius=R
  Wr [rad/s] : Outport
  Pg [W] : Outport  Port=2
  TSR [-] : Outport  Port=3
  wires:
  [TSR] -> AerodynamicTorque1/3
  beta [rad]/1 -> [beta]
  Constant/1 -> Divide/2
  V [m/s]/1 -> [V], AerodynamicTorque1/2
  [beta] -> Cpqt lookup1/2
  Cpqt lookup1/1 -> AerodynamicTorque1/1
  Divide/1 -> Discrete-Time Integrator/1  "omegar_dot"
  Discrete-Time Integrator/1 -> [Wr], TSR1/1
  AerodynamicTorque1/1 -> [Tr], Sum/1
  Sum/1 -> Divide/1
  TSR1/1 -> Cpqt lookup1/1, [TSR]
  [V] -> TSR1/2
  [Wg] -> Product/2
  Product/1 -> Pg [W]/1
  [Tg] -> Product/1
  [Wr] -> Wr [rad/s]/1
  [TSR] -> TSR [-]/1
  Sum1/1 -> Sum/2
  [Wr] -> Sum2/1
  [Wg] -> Gain7/1
  Sum2/1 -> Discrete-Time Integrator1/1  "theta_s_dot"
  Discrete-Time Integrator1/1 -> [thetas]
  [thetas] -> Gain/1
  Gain/1 -> Sum1/2
  [Wr] -> Gain2/1
  Gain2/1 -> Sum1/1
  [Wg] -> Gain8/1
  Gain3/1 -> Sum1/3
  Gain6/1 -> Sum4/3
  [thetas] -> Gain4/1
  Gain5/1 -> Sum4/1
  Gain4/1 -> Sum4/2
  Sum3/1 -> Divide1/1
  Divide1/1 -> Discrete-Time Integrator2/1  "omegarg_dot"
  Discrete-Time Integrator2/1 -> Gain12/1
  Gain7/1 -> Sum2/2
  Gain8/1 -> Gain3/1
  [Wg] -> Gain11/1
  Constant1/1 -> Gain9/1
  Tg [Nm]/1 -> Gain10/1, [Tg]
  [Wr] -> Gain5/1
  Gain10/1 -> Sum3/1
  Gain11/1 -> Gain6/1
  Sum4/1 -> Sum3/2
  Gain9/1 -> Divide1/2
  Gain12/1 -> [Wg]

== matlab function DRC_SimulinkLibrary/TSR_OptimalRotorSpeed/Optimal rotor speed ==
  data: u input size=[1 3]; Wr_opt output
function Wr_opt = fcn(u)
    Wr_opt = tsr(u(1), u(2), u(3), 'WR');
end

== matlab function DRC_SimulinkLibrary/TSR/TSR ==
  data: u input size=[1 3]; tsr_out output
function tsr_out = fcn(u)
    tsr_out = tsr(u(1), u(2), u(3));
end

== matlab function DRC_SimulinkLibrary/AerodynamicTorque/AerodynamicTorqueEstimate ==
  data: rho input; R input; Cp input; T output; V input; TSR input
function T = aerodynamictorque(rho, R, Cp, V, TSR)

T = aerodynamictorque(rho, R, Cp, V, TSR);

== matlab function DRC_SimulinkLibrary/FirstOrderHighPassFilter/HighPassFilter ==
  data: u input; y output; wc input; reset input; resetValue input; Ts input
function y = fcn(u, wc, reset, resetValue, Ts)

    persistent u_prev1 y_prev1
    K = 2.0/Ts; % Constant gain
    
    if isempty(u_prev1) || reset
        u_prev1 = resetValue; % Initialize persistent input signal variable
        y_prev1 = resetValue; % Initialize persistent output signal variable
        
        y = resetValue;
    else
        y = K/(wc + K)*u - K/(wc + K)*u_prev1 - (wc - K)/(wc + K)*y_prev1;
        
        u_prev1 = u;
        y_prev1 = y;
    end

end

== matlab function DRC_SimulinkLibrary/FirstOrderLowPassFilter/First-order low-pass filter ==
  data: u input; wc input; reset input; resetValue input; y output; Ts input
function y = FirstLPF(u, wc, reset, resetValue, Ts)

    persistent y_prev1 u_prev1

    if isempty(u_prev1) || reset
        y_prev1 = resetValue;
        u_prev1 = resetValue;
        
        y = resetValue;
    else
        y = (Ts*wc*u + Ts*wc*u_prev1 - (Ts*wc-2.0)*y_prev1)/(Ts*wc+2.0);

        u_prev1 = u;
        y_prev1 = y;
    end

end

== matlab function DRC_SimulinkLibrary/Subsystem1/MATLAB Function ==
  data: u input; y output; u_init input
function y = firstsampleinit(u, u_init)

persistent y_last

if isempty(y_last)
    y = u_init;    
else
    y = u;
end

y_last = y;

== matlab function DRC_SimulinkLibrary/SecondOrderLowPassFilter/Second-order low-pass filter ==
  data: u input; wn input; Damp input; y output; Ts input
function y = SecLPF(u, wn, Damp, Ts)

persistent y_prev1 y_prev2 u_prev1 u_prev2

if isempty(u_prev1)
    y_prev1 = u;
    y_prev2 = u;
    u_prev1 = u;
    u_prev2 = u;
end

y = 1/(4+4*Ts*Damp*wn+Ts^2*wn^2) * ( (8-2*Ts^2*wn^2)*y_prev1 + ...
    (-4+4*Ts*Damp*wn-Ts^2*wn^2)*y_prev2 + (Ts^2*wn^2)*u ...
    + (2*Ts^2*wn^2)*u_prev1 + (Ts^2*wn^2)*u_prev2 );

u_prev2   = u_prev1;
u_prev1   = u;
y_prev2  = y_prev1;
y_prev1  = y;

== matlab function DRC_SimulinkLibrary/PISaturation/MATLAB Function ==
  data: error input; saturationDirection output; kp input
function saturationDirection = fcn(error, kp)
% This function detects whether the control signal direction is towards a
% saturation boundary (true, 1) or in the desaturation direction.

    signError = sign(error);
    signGain = sign(kp*error);

    saturationDirection = signError*signGain;
end

== matlab function DRC_SimulinkLibrary/MATLAB Function ==
  data: A input; clockPeriod input; y output size=1
function y = RBS(A, clockPeriod)

persistent counter yprev

if isempty(yprev)
    yprev = 0;
    counter = clockPeriod;
end

randomNumber = rand(1) - 0.5;

if counter >= clockPeriod
    if randomNumber <= 0
        out = -A;
    else
        out = A;
    end
    
    yprev = out;
    counter = 0;
else
    out = yprev;
end

counter = counter + 1;

y = out;

== matlab function DRC_SimulinkLibrary/NotchFilter/MATLAB Function ==
  data: u input; betaNumDen input; wn input; y output; Ts input; reset input; resetValue input
function y = NotchFilter(u, betaNumDen, wn, Ts, reset, resetValue)

persistent u_prev1 u_prev2 y_prev1 y_prev2
if isempty(u_prev1) || reset
    u_prev1 = resetValue;
    u_prev2 = resetValue;
    y_prev1 = resetValue;
    y_prev2 = resetValue;
    
    y = resetValue;
elseif any([betaNumDen(1) betaNumDen(2) wn] == 0)
    y = u;
else
    % Prepare filter elements from current input
    K = 2/Ts;
    Part1 = (K^2 + 2*wn*betaNumDen(1) * K + wn^2) / (K^2 + 2*wn*betaNumDen(2) * K + wn^2);
    Part2 = (2 * wn^2 - 2 * K^2)  / (K^2 + 2*wn*betaNumDen(2) * K + wn^2);
    Part3 = (K^2 - 2*wn*betaNumDen(1) * K + wn^2) / (K^2 + 2*wn*betaNumDen(2) * K + wn^2);
    Part4 = (2 * wn^2 - 2 * K^2)  / (K^2 + 2*wn*betaNumDen(2) * K + wn^2);
    Part5 = (K^2 - 2*wn*betaNumDen(2)* K + wn^2)/ (K^2 + 2*wn*betaNumDen(2) * K + wn^2);
    
    % Compute filter output
    y = Part1*u + Part2*u_prev1 + Part3*u_prev2 - Part4*y_prev1 - Part5*y_prev2;
    
    % Save signals for next time step
    u_prev2 = u_prev1;
    u_prev1 = u;
    
    y_prev2 = y_prev1;
    y_prev1 = y;
end

end
